simulink model "Enceinte_simple"  (R2025b)
settings: Solver=VariableStepAuto  StartTime=0.0  StopTime=10.0  RelTol=1e-3
settings Model: Creator=elio  LastModifiedBy=elio

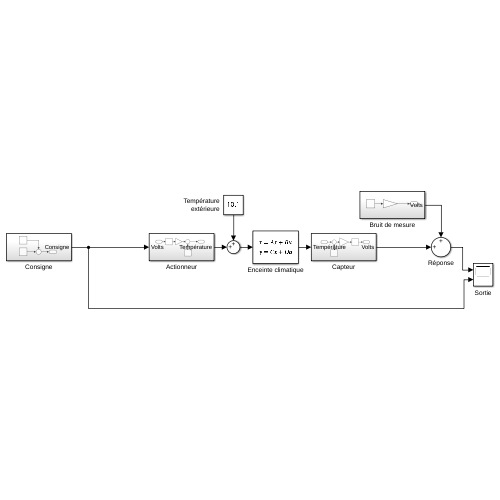
[thumbnail: Simulink's stored preview of the top-level diagram]
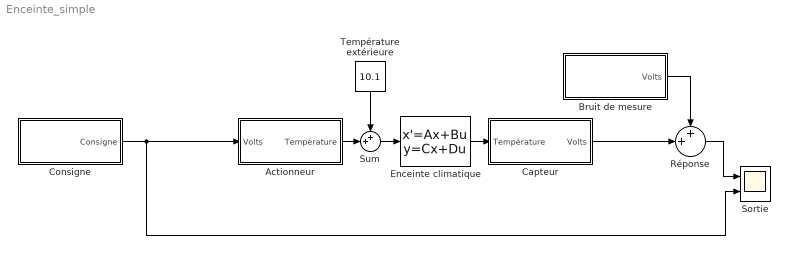
== system Enceinte_simple ==
  Actionneur : Subsystem
  Bruit de mesure : Subsystem
  Capteur : Subsystem
  Consigne : Subsystem
  Enceinte climatique : StateSpace  A=-2  B=2  D=0  InitialCondition=9.95
  Réponse : Sum  Inputs=++|
  Sortie : Scope  NumInputPorts=2
      settings: ActiveDisplayYMinimum=-0.32845703124999925  ActiveDisplayYMaximum=3.9662695312499996
  Sum : Sum  Inputs=++|
  Température extérieure : Constant  Value=10.1
  wires:
  Enceinte climatique/1 -> Capteur/1(Température)
  Actionneur/1(Température) -> Sum/2
  Sum/1 -> Enceinte climatique/1
  Température extérieure/1 -> Sum/1
  Consigne/1(Consigne) -> Sortie/2, Actionneur/1(Volts)
  Capteur/1(Volts) -> Réponse/2
  Réponse/1 -> Sortie/1
  Bruit de mesure/1(Volts) -> Réponse/1

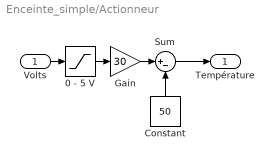
== system Enceinte_simple/Actionneur ==
  Volts : Inport
  "0 - 5 V " : Saturate  UpperLimit=5  LowerLimit=0
  Constant : Constant  Value=50
  Gain : Gain  Gain=30
  Sum : Sum  Inputs=|+-
  Température : Outport
  wires:
  Volts/1 -> "0 - 5 V "/1
  "0 - 5 V "/1 -> Gain/1
  Gain/1 -> Sum/1
  Constant/1 -> Sum/2
  Sum/1 -> Température/1

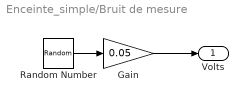
== system Enceinte_simple/Bruit de mesure ==
  Gain : Gain  Gain=0.05
  Random Number : RandomNumber  Variance=0.5  SampleTime=0.01
  Volts : Outport
  wires:
  Random Number/1 -> Gain/1
  Gain/1 -> Volts/1

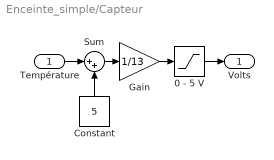
== system Enceinte_simple/Capteur ==
  Température : Inport
  "0 - 5 V " : Saturate  UpperLimit=5  LowerLimit=0
  Constant : Constant  Value=5
  Gain : Gain  Gain=1/13
  Sum : Sum  Inputs=|++
  Volts : Outport
  wires:
  Constant/1 -> Sum/2
  Température/1 -> Sum/1
  Sum/1 -> Gain/1
  Gain/1 -> "0 - 5 V "/1
  "0 - 5 V "/1 -> Volts/1

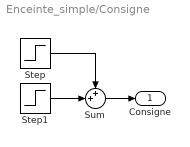
== system Enceinte_simple/Consigne ==
  Step : Step  Time=4  After=-0.5  SampleTime=0.01
  Step1 : Step  Time=0.5  Before=1.66  After=2.33  SampleTime=0.01
  Sum : Sum  Inputs=++|
  Consigne : Outport
  wires:
  Step/1 -> Sum/1
  Step1/1 -> Sum/2
  Sum/1 -> Consigne/1
